simulink model "experiment5"  (R2020b)
settings: Solver=VariableStepAuto  StartTime=0.0  StopTime=10.0  RelTol=1e-3
settings Model: Creator=LENOVO  LastModifiedBy=LENOVO

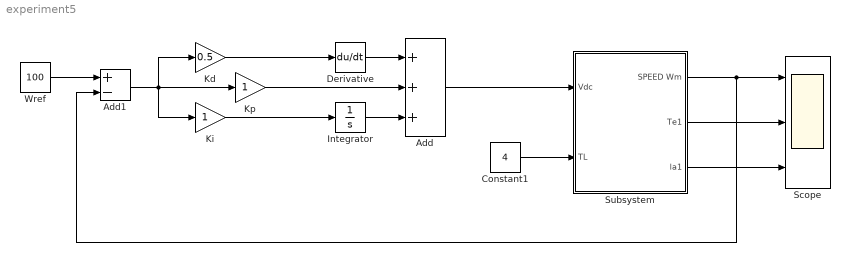
== system experiment5 ==
  Add : Sum  Inputs=+++
  Add1 : Sum  Inputs=+-
  Constant1 : Constant  Value=4
  Derivative : Derivative
  Integrator : Integrator
  Kd : Gain  Gain=0.5
  Ki : Gain
  Kp : Gain
  Scope : Scope  NumInputPorts=3
  Subsystem : Subsystem
  Wref : Constant  Value=100
  wires:
  Constant1/1 -> Subsystem/2(TL)
  Subsystem/2(Te1) -> Scope/2
  Subsystem/3(la1) -> Scope/3
  Add/1 -> Subsystem/1(Vdc)
  Integrator/1 -> Add/3
  Derivative/1 -> Add/1
  Kd/1 -> Derivative/1
  Kp/1 -> Add/2
  Ki/1 -> Integrator/1
  Add1/1 -> Ki/1, Kd/1, Kp/1
  Subsystem/1(SPEED Wm) -> Add1/2, Scope/1
  Wref/1 -> Add1/1

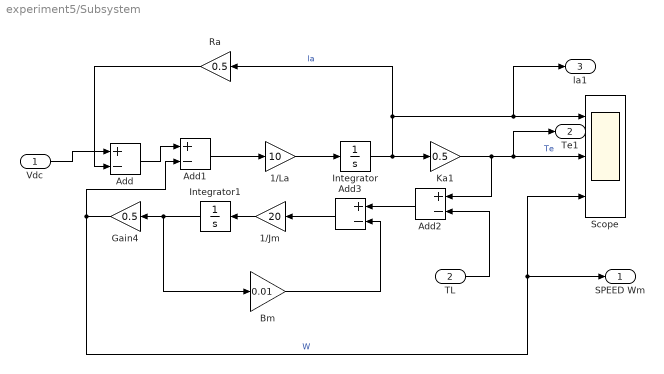
== system experiment5/Subsystem ==
  Vdc : Inport
  TL : Inport  Port=2
  1/Jm : Gain  Gain=20
  1/La : Gain  Gain=10
  Add{,1..3} (4 alike) : Sum  Inputs=+-
  Bm : Gain  Gain=0.01
  Gain4 : Gain  Gain=0.5
  Integrator : Integrator
  Integrator1 : Integrator
  Ka1 : Gain  Gain=0.5
  Ra : Gain  Gain=0.5
  Scope : Scope  NumInputPorts=3
  SPEED Wm : Outport
  Te1 : Outport  Port=2
  la1 : Outport  Port=3
  wires:
  Ra/1 -> Add/2
  Add2/1 -> Add3/1
  Gain4/1 -> SPEED Wm/1, Scope/3, Add1/2  "W"
  Integrator/1 -> Ra/1, la1/1, Scope/1, Ka1/1  "la"
  Vdc/1 -> Add/1
  Integrator1/1 -> Bm/1, Gain4/1
  TL/1 -> Add2/2
  Ka1/1 -> Add2/1, Te1/1, Scope/2  "Te"
  Add/1 -> Add1/1
  Add3/1 -> 1/Jm/1
  Bm/1 -> Add3/2
  1/La/1 -> Integrator/1
  Add1/1 -> 1/La/1
  1/Jm/1 -> Integrator1/1
